simulink model "logicGate"  (Simulink 7.1)
settings: Solver=ode1  StartTime=0.0  StopTime=10.0  FixedStep=1  RelTol=1e-3
libraries: simulink x1
settings Model: Creator=Osmaz  LastModifiedBy=Osmaz
settings OptimizationCC: ExpressionDepthLimit=128  InitFltsAndDblsToZero=off
settings DebuggingCC: SolverPrmCheckMsg=none  FcnCallInpInsideContextMsg=Enable All  StateNameClashWarn=none  StrictBusMsg=ErrorLevel1
settings CodeAppCC: CustomSymbolStrType=$N$R$M_T
settings GRTTargetCC: TargetFunctionLibrary=C89/C90 (ANSI)  CPPClassGenCompliant=off

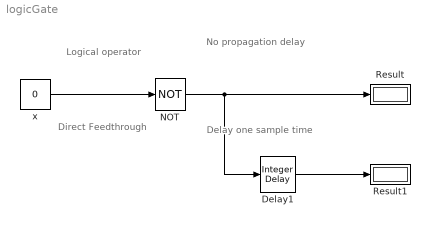
== system logicGate ==
  note: Direct Feedthrough
  note: Delay one sample time
  note: Logical operator
  note: No propagation delay
  Delay1 : simulink/Discrete/Integer Delay  NumDelays=1  vinit=0  samptime=-1
  NOT : Logic  Operator=NOT  IconShape=distinctive  AllPortsSameDT=off  OutDataTypeStr=boolean  OutDataTypeMode=boolean
  Result : Display
  Result1 : Display
  x : Constant  Value=0  OutMin=-8  OutMax=7  OutDataTypeStr=int8  SampleTime=1  OutDataTypeMode=int8
  wires:
  NOT/1 -> Delay1/1, Result/1
  x/1 -> NOT/1
  Delay1/1 -> Result1/1
